simulink model "Simulink_20_10_1"  (R2020a)
settings: Solver=VariableStepAuto  StartTime=0.0  StopTime=75  RelTol=1e-3
values from neighbouring files (symbols this model uses):
  K_REI = [Ks(:,1) Ks(:,2)]    [Retro_Alimentacion_Integral.m]    (also in Workspace_20_Octubre.mat = [18.874405068 -8.29205202847 -9.96547850829 -1.40770716274]; Workspace_21_Octubre.mat = [34.4760176193 -15.5235439726 -4.32287066177 -1.41201865408])
  Ki_REI = -Ks(:,3)    [Retro_Alimentacion_Integral.m]    (also in Workspace_20_Octubre.mat = 7.05565296496; Workspace_21_Octubre.mat = 13.3109774254)
undefined symbols (not defined in the file or in its folder): Grua_ss
settings Model: Creator=geral  LastModifiedBy=geral

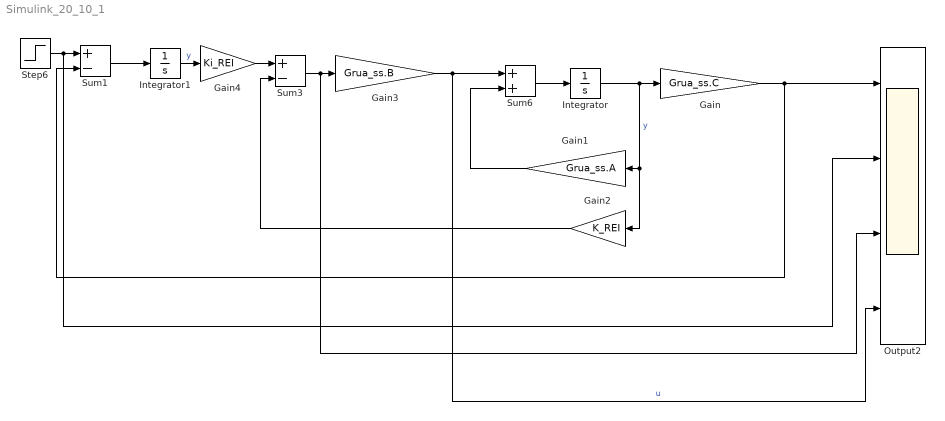
== system Simulink_20_10_1 ==
  Gain : Gain  Gain=Grua_ss.C
  Gain1 : Gain  Gain=Grua_ss.A
  Gain2 : Gain  Gain=K_REI
  Gain3 : Gain  Gain=Grua_ss.B
  Gain4 : Gain  Gain=Ki_REI
  Integrator : Integrator
  Integrator1 : Integrator
  Output2 : Scope  NumInputPorts=4
  Step6 : Step  Time=0.1  After=0.5  SampleTime=0
  Sum1 : Sum  Inputs=+-
  Sum3 : Sum  Inputs=+-
  Sum6 : Sum
  wires:
  Sum6/1 -> Integrator/1
  Gain3/1 -> Output2/4, Sum6/1  "u"
  Sum3/1 -> Output2/3, Gain3/1
  Integrator/1 -> Gain2/1, Gain1/1, Gain/1  "y"
  Gain1/1 -> Sum6/2
  Integrator1/1 -> Gain4/1  "y"
  Gain4/1 -> Sum3/1
  Gain2/1 -> Sum3/2
  Sum1/1 -> Integrator1/1
  Gain/1 -> Output2/1, Sum1/2
  Step6/1 -> Output2/2, Sum1/1
